simulink model "W02_G_derivative_bench"  (R2024b)
settings: Solver=ode4  StartTime=0  StopTime=bench_T  FixedStep=h  RelTol=1e-3
values from neighbouring files (symbols this model uses):
  bench_noise = 0.005    [W02_0_setup.m]
  bench_w = 0.5    [W02_0_setup.m]
  Nf = 20    [W02_0_setup.m]    (also in W02_G_lowpass_filter.m = Nf(i))
  noise_ts = 0.01    [W02_0_setup.m]
settings Model: Creator=admin  LastModifiedBy=admin
settings DataIOCC: ReturnWorkspaceOutputs=off

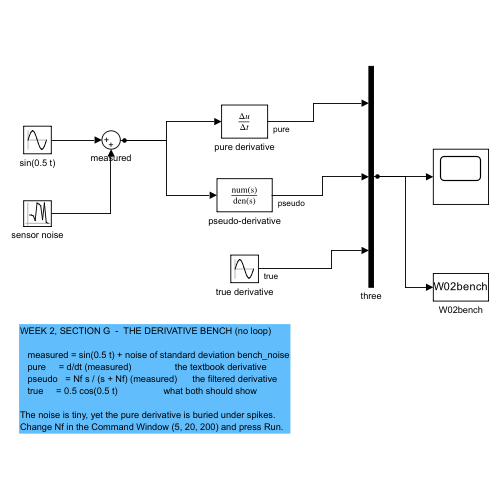
[thumbnail: Simulink's stored preview of the top-level diagram]
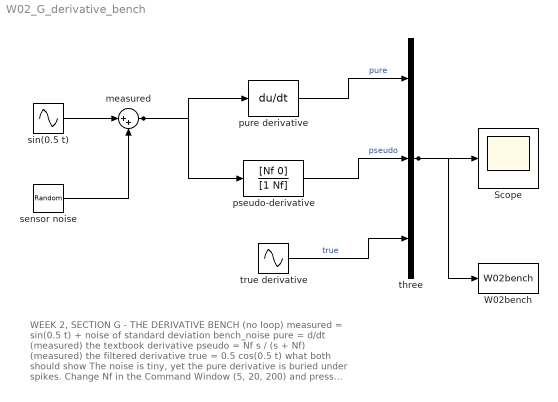
== system W02_G_derivative_bench ==
  note: WEEK 2, SECTION G  -  THE DERIVATIVE BENCH (no loop)
      |
      |    measured = sin(0.5 t) + noise of standard deviation bench_noise
      |    pure     = d/dt (measured)                 the textbook derivative
      |    pseudo   = Nf s / (s + Nf) (measured)      the filtered derivative
      |    true     = 0.5 cos(0.5 t)                  what both should show
      |
      | The noise is tiny, yet the pure derivative is buried under spikes.
      | Change Nf in the Command Window (5, 20, 200) and press Run.
  Scope : Scope
  W02bench : ToWorkspace  VariableName=W02bench  SaveFormat=Structure With Time  SampleTime=-1
  measured : Sum  Inputs=|++
  pseudo-derivative : TransferFcn  Numerator=[Nf 0]  Denominator=[1 Nf]
  pure derivative : Derivative
  sensor noise : RandomNumber  Variance=bench_noise^2  Seed=23341  SampleTime=noise_ts
  sin(0.5 t) : Sin  Frequency=bench_w  SampleTime=0
  three : Mux  Inputs=3
  true derivative : Sin  Amplitude=bench_w  Frequency=bench_w  Phase=pi/2  SampleTime=0
  wires:
  sin(0.5 t)/1 -> measured/1
  sensor noise/1 -> measured/2
  measured/1 -> pure derivative/1, pseudo-derivative/1
  pure derivative/1 -> three/1  "pure"
  pseudo-derivative/1 -> three/2  "pseudo"
  true derivative/1 -> three/3  "true"
  three/1 -> Scope/1, W02bench/1
